simulink model "airdropx_mpc_closed_loop_tuned"  (R2024b)
settings: Solver=FixedStepDiscrete  StartTime=0.0  StopTime=airdropx_stop_time_s  FixedStep=dt  RelTol=1e-3
PreLoadFcn:
  | airdropx_mpc_setup_closed_loop_workspace('Model','airdropx_mpc_closed_loop_tuned');
PostLoadFcn:
  | airdropx_mpc_setup_closed_loop_workspace('Model','airdropx_mpc_closed_loop_tuned');
InitFcn:
  | airdropx_mpc_setup_closed_loop_workspace('Model','airdropx_mpc_closed_loop_tuned');
values from neighbouring files (symbols this model uses):
  dt = median(diff(unique(t)), "omitnan")    [airdropx_mpc_assess_identification.m]    (also in airdropx_mpc_controller.m = 0.1; airdropx_mpc_nominal_model.m = cfg.dt_s; airdropx_mpc_state_from_table.m = [max(tg(2) - tg(1), eps); max(diff(tg), eps)]; sfun_airdropx_mpc_controller.m = max(t - data.prev_t, eps))
undefined symbols (not defined in the file or in its folder): airdropx_ballistics_gravity_mps2, airdropx_ballistics_k_drag, airdropx_ballistics_side_wind_gain, airdropx_carp_drop_total, airdropx_carp_interval_s, airdropx_carp_min_safe_alt_m, airdropx_carp_release_window_s, airdropx_carp_target_e_m, airdropx_carp_target_n_m, airdropx_fixed_drop_interval_s, airdropx_fixed_drop_pulse_s, airdropx_fixed_drop_start_s, airdropx_fixed_drop_total, airdropx_initial_drop_cmd, airdropx_initial_elevator_delta, airdropx_initial_throttle_cmd, airdropx_reset_cmd, airdropx_wind_dir_from_deg, airdropx_wind_speed_mps
libraries: vrlib x1
settings Model: Creator=qq263  LastModifiedBy=qq263

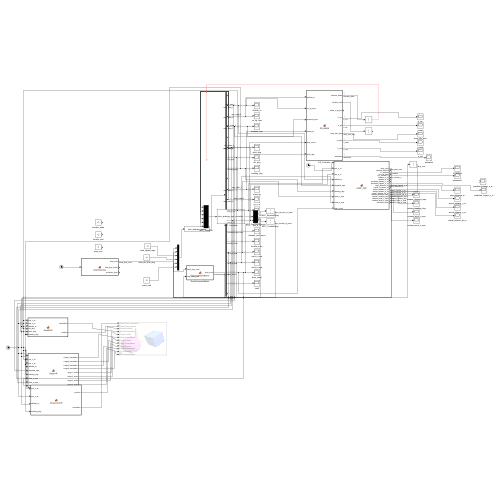
[thumbnail: Simulink's stored preview of the top-level diagram]
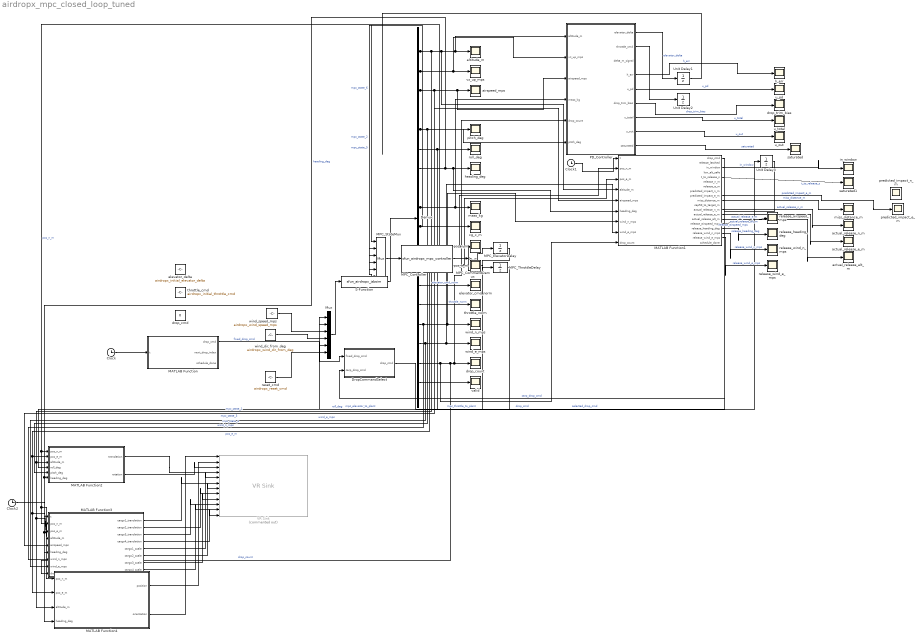
== system airdropx_mpc_closed_loop_tuned ==
  Clock : Clock
  Clock1 : Clock
  Clock2 : Clock
  Demux : Demux  Outputs=20
  DropCommandSelect : MATLAB Function  TreatAsAtomicUnit=on
  MATLAB Function : MATLAB Function  TreatAsAtomicUnit=on
  MATLAB Function1 : MATLAB Function  TreatAsAtomicUnit=on
  MATLAB Function2 : MATLAB Function  TreatAsAtomicUnit=on
  MATLAB Function3 : MATLAB Function  TreatAsAtomicUnit=on
  MATLAB Function4 : MATLAB Function  TreatAsAtomicUnit=on
  MPC_CommandDemux : Demux  Outputs=2
  MPC_Controller : M-S-Function  FunctionName=sfun_airdropx_mpc_controller  Parameters=''
  MPC_ElevatorDelay : UnitDelay  InitialCondition=airdropx_initial_elevator_delta  SampleTime=dt  HasFrameUpgradeWarning=on
  MPC_StateMux : Mux  Inputs=6
  MPC_ThrottleDelay : UnitDelay  InitialCondition=airdropx_initial_throttle_cmd  SampleTime=dt  HasFrameUpgradeWarning=on
  Mux : Mux  Inputs=6
  "PD_Controller " : MATLAB Function  TreatAsAtomicUnit=on
  S-Function : S-Function  FunctionName=sfun_airdropx_jsbsim  Parameters=projectRoot, aircraftName, icName, dt  SFunctionDeploymentMode=off  EnableBusSupport=off
  Unit Delay1 : UnitDelay  InitialCondition=airdropx_initial_elevator_delta  SampleTime=dt  HasFrameUpgradeWarning=on
  Unit Delay2 : UnitDelay  InitialCondition=airdropx_initial_throttle_cmd  SampleTime=dt  HasFrameUpgradeWarning=on
  Unit Delay3 : UnitDelay  InitialCondition=airdropx_initial_drop_cmd  SampleTime=dt  HasFrameUpgradeWarning=on
  VR Sink : vrlib/VR Sink  Commented=on  InstantiateOnLoad=on  SampleTime=0.1  ViewEnable=on  RemoteChange=off  RemoteView=off  FieldsWritten=ChaseView.orientation.4.1.1.double#ChaseView.position.3.1.1.double#Aircraft.rotation.4.1.1.double#Aircraft.translation.3.1.1.double#Cargo1.scale.3.1.1.double#Cargo1.translation.3.1.1.double#Cargo2.scale.3.1.1.double#Cargo2.translation.3.1.1.double#Cargo3.scale.3.1.1.double#Cargo3.translation.3.1.1.double#Cargo4.scale.3.1.1.double#Cargo4.translation.3.1.1.double  WorldFileName=vr\airdropx_scene.wrl  WorldDescription=AirdropX Simulink 3D Animation Scene  AutoView=on  VideoDimensions=[]  AllowVariableSize=off  FigureProperties="{'Position', 'Name', 'Viewpoint', 'CameraBound', 'CameraDirection', 'CameraPosition', 'CameraUpVector', 'ZoomFactor', 'Antialiasing', 'Headlight', 'Lighting', 'Sound', 'StatusBar', 'Stereo3D', 'Stereo3DCameraOffset', 'Stereo3DHIT', 'ToolBar', 'Textures', 'Transparency', 'Triad', 'Wireframe', 'NavZones', 'NavMode', 'NavSpeed', 'CaptureFileFormat', 'CaptureFileName', 'Record2DCompressMethod', 'Record2DCompressQuality', 'Record2D', 'Record2DFileName', 'Record2DFPS', 'NavPanel'; [2.2500000000000000e+02   1.8919999999999993e+02   1.5392000000000000e+03   7.4280000000000007e+02], 'AirdropX Simulink 3D Animation Scene', 'Auto Chase', 'on', [-1.5245731489728184e-01   1.1145762937492740e-01  -9.8200507330073861e-01], [8.3794000317414088e+01  -8.2566278091214883e+01   4.6192914514757570e+02], [2.6955468538304983e-01   9.6063863984382492e-01   6.7183891127693351e-02], [1.0000000000000000e+00], 'on', 'on', 'on', 'on', 'on', 'off', [1.0000000149011612e-01], [0.0000000000000000e+00], 'on', 'on', 'on', 'none', 'off', 'off', 'examine', 'normal', 'tif', '%f_anim_%n.tif', 'auto', [7.5000000000000000e+01], 'off', '%f_anim_%n.avi', 'auto', 'halfbar'}"
  actual_release_alt_m : Scope
  actual_release_e_m : Scope
  actual_release_n_m : Scope
  airspeed_mps : Scope
  altitude_m : Scope
  cg_x_m : Scope
  drop_cmd : Constant  Value=0
  drop_count : Scope
  drop_trim_bias : Scope
  elevator_cmd_norm : Scope
  elevator_delta : Constant  Value=airdropx_initial_elevator_delta
  h_err : Scope
  heading_deg : Scope
  in_window : Scope
  mass_kg : Scope
  "miss_distance_m " : Scope
  pitch_deg : Scope
  pos_e_m : Scope
  pos_n_m : Scope
  predicted_impact_e_m : Scope
  predicted_impact_n_m : Scope
  release_airspeed_mps : Scope
  release_heading_deg : Scope
  release_wind_e_mps : Scope
  release_wind_n_mps : Scope
  reset_cmd : Constant  Value=airdropx_reset_cmd
  roll_deg : Scope
  saturated : Scope
  saturated1 : Scope
  throttle_cmd : Constant  Value=airdropx_initial_throttle_cmd
  throttle_norm : Scope
  u_out : Scope
  u_pd : Scope
  u_total : Scope
  valid : Scope
  vz_up_mps : Scope
  wind_dir_from_deg : Constant  Value=airdropx_wind_dir_from_deg
  wind_e_mps : Scope
  wind_n_mps : Scope
  wind_speed_mps : Constant  Value=airdropx_wind_speed_mps
  wires:
  wind_speed_mps/1 -> Mux/3
  wind_dir_from_deg/1 -> Mux/4
  reset_cmd/1 -> Mux/6
  Mux/1 -> S-Function/1
  S-Function/1 -> Demux/1
  Demux/3 -> "PD_Controller "/2(vz_up_mps), vz_up_mps/1, MPC_StateMux/2  "mpc_state_2"
  Demux/4 -> MATLAB Function1/5(airspeed_mps), MATLAB Function3/5(airspeed_mps), "PD_Controller "/3(airspeed_mps), airspeed_mps/1, MPC_StateMux/3  "mpc_state_3"
  Demux/6 -> MATLAB Function2/5(pitch_deg), pitch_deg/1, "PD_Controller "/6(pitch_deg), MPC_StateMux/4  "mpc_state_4"
  Demux/19 -> valid/1
  Demux/10 -> "PD_Controller "/4(mass_kg), mass_kg/1, MPC_StateMux/5  "mpc_state_5"
  "PD_Controller "/1(elevator_delta) -> Unit Delay1/1  "elevator_delta"
  "PD_Controller "/2(throttle_cmd) -> Unit Delay2/1
  Demux/15 -> throttle_norm/1  "throttle_norm"
  Demux/14 -> elevator_cmd_norm/1  "elevator_cmd_norm"
  Demux/2 -> MATLAB Function4/3(altitude_m), MATLAB Function3/4(altitude_m), MATLAB Function2/3(altitude_m), MATLAB Function1/4(altitude_m), "PD_Controller "/1(altitude_m), altitude_m/1, MPC_StateMux/1  "mpc_state_1"
  Unit Delay1/1 -> ?
  Demux/18 -> MATLAB Function1/9(drop_count), MATLAB Function3/9(drop_count), "PD_Controller "/5(drop_count), drop_count/1  "drop_count"
  Clock/1 -> MATLAB Function/1(t)
  Clock1/1 -> MATLAB Function1/1(t)
  Demux/12 -> MATLAB Function4/1(pos_n_m), MATLAB Function3/2(pos_n_m), MATLAB Function2/1(pos_n_m), MATLAB Function1/2(pos_n_m), pos_n_m/1  "pos_n_m"
  Demux/13 -> MATLAB Function4/2(pos_e_m), MATLAB Function3/3(pos_e_m), MATLAB Function2/2(pos_e_m), MATLAB Function1/3(pos_e_m), pos_e_m/1  "pos_e_m"
  Demux/16 -> MATLAB Function3/7(wind_n_mps), MATLAB Function1/7(wind_n_mps), wind_n_mps/1  "wind_n_mps"
  Demux/17 -> MATLAB Function3/8(wind_e_mps), MATLAB Function1/8(wind_e_mps), wind_e_mps/1  "wind_e_mps"
  Demux/8 -> MATLAB Function4/4(heading_deg), MATLAB Function3/6(heading_deg), MATLAB Function2/6(heading_deg), MATLAB Function1/6(heading_deg), heading_deg/1  "heading_deg"
  Demux/11 -> cg_x_m/1, MPC_StateMux/6  "mpc_state_6"
  "PD_Controller "/4(h_err) -> h_err/1  "h_err"
  "PD_Controller "/5(u_pd) -> u_pd/1  "u_pd"
  "PD_Controller "/6(drop_trim_bias) -> drop_trim_bias/1  "drop_trim_bias"
  "PD_Controller "/7(u_total) -> u_total/1  "u_total"
  "PD_Controller "/8(u_out) -> u_out/1  "u_out"
  "PD_Controller "/9(saturated) -> saturated/1  "saturated"
  MATLAB Function1/5(t_to_release_s) -> saturated1/1  "t_to_release_s"
  MATLAB Function1/3(in_window) -> in_window/1  "in_window"
  MATLAB Function1/10(miss_distance_m) -> "miss_distance_m "/1  "miss_distance_m"
  MATLAB Function1/12(actual_release_n_m) -> actual_release_n_m/1  "actual_release_n_m"
  MATLAB Function1/13(actual_release_e_m) -> actual_release_e_m/1  "actual_release_e_m"
  MATLAB Function1/14(actual_release_alt_m) -> actual_release_alt_m/1  "actual_release_alt_m"
  MATLAB Function1/9(predicted_impact_e_m) -> predicted_impact_e_m/1  "predicted_impact_e_m"
  MATLAB Function1/15(release_airspeed_mps) -> release_airspeed_mps/1  "release_airspeed_mps"
  MATLAB Function1/16(release_heading_deg) -> release_heading_deg/1  "release_heading_deg"
  MATLAB Function1/17(release_wind_n_mps) -> release_wind_n_mps/1  "release_wind_n_mps"
  MATLAB Function1/18(release_wind_e_mps) -> release_wind_e_mps/1  "release_wind_e_mps"
  Demux/7 -> MATLAB Function2/4(roll_deg), roll_deg/1  "roll_deg"
  Clock2/1 -> MATLAB Function3/1(t)
  MATLAB Function2/2(rotation) -> VR Sink/3
  MATLAB Function2/1(translation) -> VR Sink/4
  MATLAB Function3/5(cargo1_scale) -> VR Sink/5
  MATLAB Function3/1(cargo1_translation) -> VR Sink/6
  MATLAB Function3/6(cargo2_scale) -> VR Sink/7
  MATLAB Function3/2(cargo2_translation) -> VR Sink/8
  MATLAB Function3/7(cargo3_scale) -> VR Sink/9
  MATLAB Function3/3(cargo3_translation) -> VR Sink/10
  MATLAB Function3/8(cargo4_scale) -> VR Sink/11
  MATLAB Function3/4(cargo4_translation) -> VR Sink/12
  MATLAB Function4/1(position) -> VR Sink/2
  MATLAB Function4/2(orientation) -> VR Sink/1
  MATLAB Function/1(drop_cmd) -> DropCommandSelect/1(fixed_drop_cmd)  "fixed_drop_cmd"
  MATLAB Function1/1(drop_cmd) -> DropCommandSelect/2(carp_drop_cmd)  "carp_drop_cmd"
  DropCommandSelect/1(drop_cmd) -> Unit Delay3/1  "selected_drop_cmd"
  Unit Delay3/1 -> Mux/5  "drop_cmd"
  MPC_StateMux/1 -> MPC_Controller/1
  MPC_Controller/1 -> MPC_CommandDemux/1
  MPC_CommandDemux/1 -> MPC_ElevatorDelay/1
  MPC_CommandDemux/2 -> MPC_ThrottleDelay/1
  MPC_ElevatorDelay/1 -> Mux/1  "mpc_elevator_to_plant"
  MPC_ThrottleDelay/1 -> Mux/2  "mpc_throttle_to_plant"

== matlab function airdropx_mpc_closed_loop_tuned/MATLAB Function ==
  data: t input; drop_cmd output; next_drop_index output; schedule_done output; airdropx_fixed_drop_start_s parameter; airdropx_fixed_drop_interval_s parameter; airdropx_fixed_drop_pulse_s parameter; airdropx_fixed_drop_total parameter
function [drop_cmd, next_drop_index, schedule_done] = DropSchedule(t, airdropx_fixed_drop_start_s, airdropx_fixed_drop_interval_s, airdropx_fixed_drop_pulse_s, airdropx_fixed_drop_total)
%#codegen
[drop_cmd, next_drop_index, schedule_done] = airdropx_four_drop_schedule(t, ...
    airdropx_fixed_drop_start_s, airdropx_fixed_drop_interval_s, ...
    airdropx_fixed_drop_pulse_s, airdropx_fixed_drop_total);
end

== matlab function airdropx_mpc_closed_loop_tuned/PD_Controller  ==
  data: altitude_m input; elevator_delta output; vz_up_mps input; airspeed_mps input; mass_kg input; throttle_cmd output; drop_count input; delta_m_signal output; h_err output; u_pd output; drop_trim_bias output; u_total output; u_out output; saturated output; pitch_deg input; airdropx_target_altitude_m parameter; airdropx_pd_Kp parameter; airdropx_pd_Kd parameter; airdropx_pd_u_limit parameter; airdropx_pd_u_rate_limit parameter; airdropx_pd_K_mass parameter; airdropx_pd_bias_rate_limit parameter; airdropx_pd_throttle_kp parameter; airdropx_pd_throttle_fixed parameter; airdropx_pd_throttle_alt_kp parameter; airdropx_pd_throttle_vz_kd parameter; airdropx_pd_v_ref_mps parameter; airdropx_pd_pitch_ref_deg parameter; airdropx_pd_pitch_kp parameter; airdropx_pd_pitch_limit parameter; airdropx_pd_pitch_rate_kd parameter; airdropx_pd_pitch_rate_limit parameter; airdropx_pd_dt_s parameter; airdropx_drop_mass_signal_kg parameter; airdropx_initial_elevator_delta parameter
function [elevator_delta, throttle_cmd, delta_m_signal, h_err, u_pd, drop_trim_bias, u_total, u_out, saturated] = PD_NW20(altitude_m, vz_up_mps, airspeed_mps, mass_kg, drop_count, pitch_deg, airdropx_target_altitude_m, airdropx_pd_Kp, airdropx_pd_Kd, airdropx_pd_u_limit, airdropx_pd_u_rate_limit, airdropx_pd_K_mass, airdropx_pd_bias_rate_limit, airdropx_pd_throttle_kp, airdropx_pd_throttle_fixed, airdropx_pd_throttle_alt_kp, airdropx_pd_throttle_vz_kd, airdropx_pd_v_ref_mps, airdropx_pd_pitch_ref_deg, airdropx_pd_pitch_kp, airdropx_pd_pitch_limit, airdropx_pd_pitch_rate_kd, airdropx_pd_pitch_rate_limit, airdropx_pd_dt_s, airdropx_drop_mass_signal_kg, airdropx_initial_elevator_delta)
%#codegen

[elevator_delta, throttle_cmd, delta_m_signal, h_err, u_pd, drop_trim_bias, u_total, u_out, saturated] = ...
    airdropx_pd_nw20_block(altitude_m, vz_up_mps, airspeed_mps, pitch_deg, mass_kg, drop_count, ...
        airdropx_target_altitude_m, airdropx_pd_Kp, airdropx_pd_Kd, ...
        airdropx_pd_u_limit, airdropx_pd_u_rate_limit, airdropx_pd_K_mass, ...
        airdropx_pd_bias_rate_limit, airdropx_pd_throttle_kp, ...
        airdropx_pd_throttle_fixed, airdropx_pd_throttle_alt_kp, ...
        airdropx_pd_throttle_vz_kd, airdropx_pd_v_ref_mps, ...
        airdropx_drop_mass_signal_kg, airdropx_initial_elevator_delta, ...
        airdropx_pd_pitch_ref_deg, airdropx_pd_pitch_kp, airdropx_pd_pitch_limit, ...
        airdropx_pd_pitch_rate_kd, airdropx_pd_pitch_rate_limit, airdropx_pd_dt_s);

end

== matlab function airdropx_mpc_closed_loop_tuned/MATLAB Function1 ==
  data: t input; drop_cmd output; pos_n_m input; pos_e_m input; altitude_m input; airspeed_mps input; heading_deg input; wind_n_mps input; wind_e_mps input; drop_count input; release_latched output; in_window output; low_alt_safe output; t_to_release_s output; release_n_m output; release_e_m output; predicted_impact_n_m output; predicted_impact_e_m output; miss_distance_m output; cep50_to_target_m output; actual_release_n_m output; actual_release_e_m output; actual_release_alt_m output; release_airspeed_mps output; release_heading_deg output; release_wind_n_mps output; release_wind_e_mps output; schedule_done output; airdropx_carp_target_n_m parameter; airdropx_carp_target_e_m parameter; airdropx_carp_release_window_s parameter; airdropx_carp_interval_s parameter; airdropx_carp_drop_total parameter; airdropx_carp_min_safe_alt_m parameter; airdropx_ballistics_gravity_mps2 parameter; airdropx_ballistics_k_drag parameter; airdropx_ballistics_side_wind_gain parameter
function [drop_cmd, release_latched, in_window, low_alt_safe, t_to_release_s, release_n_m, release_e_m, predicted_impact_n_m, predicted_impact_e_m, miss_distance_m, cep50_to_target_m, actual_release_n_m, actual_release_e_m, actual_release_alt_m, release_airspeed_mps, release_heading_deg, release_wind_n_mps, release_wind_e_mps, schedule_done] = CARP_CEP(t, pos_n_m, pos_e_m, altitude_m, airspeed_mps, heading_deg, wind_n_mps, wind_e_mps, drop_count, airdropx_carp_target_n_m, airdropx_carp_target_e_m, airdropx_carp_release_window_s, airdropx_carp_interval_s, airdropx_carp_drop_total, airdropx_carp_min_safe_alt_m, airdropx_ballistics_gravity_mps2, airdropx_ballistics_k_drag, airdropx_ballistics_side_wind_gain)
%#codegen

[drop_cmd, release_latched, in_window, low_alt_safe, t_to_release_s, release_n_m, release_e_m, predicted_impact_n_m, predicted_impact_e_m, miss_distance_m, cep50_to_target_m, actual_release_n_m, actual_release_e_m, actual_release_alt_m, release_airspeed_mps, release_heading_deg, release_wind_n_mps, release_wind_e_mps, schedule_done] = ...
    airdropx_carp_cep_block(t, pos_n_m, pos_e_m, altitude_m, airspeed_mps, heading_deg, ...
        wind_n_mps, wind_e_mps, drop_count, ...
        airdropx_carp_target_n_m, airdropx_carp_target_e_m, ...
        airdropx_carp_release_window_s, airdropx_carp_interval_s, ...
        airdropx_carp_drop_total, airdropx_carp_min_safe_alt_m, ...
        airdropx_ballistics_gravity_mps2, airdropx_ballistics_k_drag, ...
        airdropx_ballistics_side_wind_gain);

end

== matlab function airdropx_mpc_closed_loop_tuned/MATLAB Function2 ==
  data: pos_n_m input; translation output; pos_e_m input; altitude_m input; roll_deg input; pitch_deg input; heading_deg input; rotation output
function [translation, rotation] = AircraftVR(pos_n_m, pos_e_m, altitude_m, roll_deg, pitch_deg, heading_deg)
%#codegen
[translation, rotation] = airdropx_vr_aircraft_pose(pos_n_m, pos_e_m, altitude_m, roll_deg, pitch_deg, heading_deg);
end

== matlab function airdropx_mpc_closed_loop_tuned/MATLAB Function3 ==
  data: t input; pos_n_m input; cargo1_translation output; pos_e_m input; altitude_m input; airspeed_mps input; heading_deg input; cargo2_translation output; wind_n_mps input; wind_e_mps input; drop_count input; cargo3_translation output; cargo4_translation output; cargo1_scale output; cargo2_scale output; cargo3_scale output; cargo4_scale output; airdropx_ballistics_gravity_mps2 parameter; airdropx_ballistics_k_drag parameter
function [cargo1_translation, cargo2_translation, cargo3_translation, cargo4_translation, cargo1_scale, cargo2_scale, cargo3_scale, cargo4_scale] = CargoVR(t, pos_n_m, pos_e_m, altitude_m, airspeed_mps, heading_deg, wind_n_mps, wind_e_mps, drop_count, airdropx_ballistics_gravity_mps2, airdropx_ballistics_k_drag)
%#codegen

[cargo1_translation, cargo2_translation, cargo3_translation, cargo4_translation, cargo1_scale, cargo2_scale, cargo3_scale, cargo4_scale] = ...
    airdropx_vr_cargo_pose(t, pos_n_m, pos_e_m, altitude_m, airspeed_mps, heading_deg, ...
        wind_n_mps, wind_e_mps, drop_count, ...
        airdropx_ballistics_gravity_mps2, airdropx_ballistics_k_drag);

end

== matlab function airdropx_mpc_closed_loop_tuned/MATLAB Function4 ==
  data: pos_n_m input; position output; pos_e_m input; altitude_m input; heading_deg input; orientation output
function [position, orientation] = ChaseViewVR(pos_n_m, pos_e_m, altitude_m, heading_deg)
%#codegen
[position, orientation] = airdropx_vr_chase_view(pos_n_m, pos_e_m, altitude_m, heading_deg);
end

== matlab function airdropx_mpc_closed_loop_tuned/DropCommandSelect ==
  data: fixed_drop_cmd input; drop_cmd output; carp_drop_cmd input; airdropx_drop_mode parameter
function drop_cmd = DropCommandSelect(fixed_drop_cmd, carp_drop_cmd, airdropx_drop_mode)
%#codegen
if airdropx_drop_mode >= 1.5
    drop_cmd = carp_drop_cmd;
else
    drop_cmd = fixed_drop_cmd;
end
end
